simulink model "PAMtesting_draft1"  (R2023a)
settings: Solver=VariableStepAuto  StartTime=0.0  StopTime=inf  RelTol=1e-3
libraries: sldrtlib x4
settings Model: Creator=Siril TD  LastModifiedBy=Siril TD

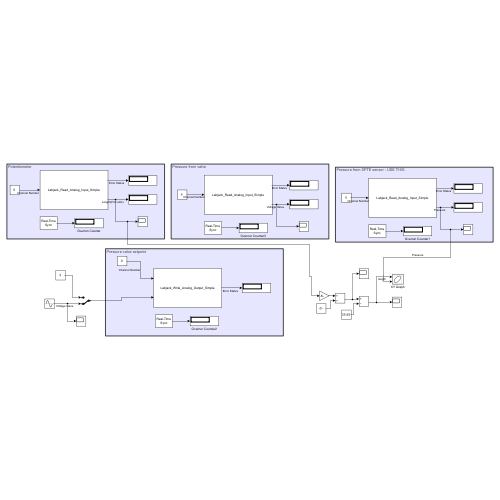
[thumbnail: Simulink's stored preview of the top-level diagram]
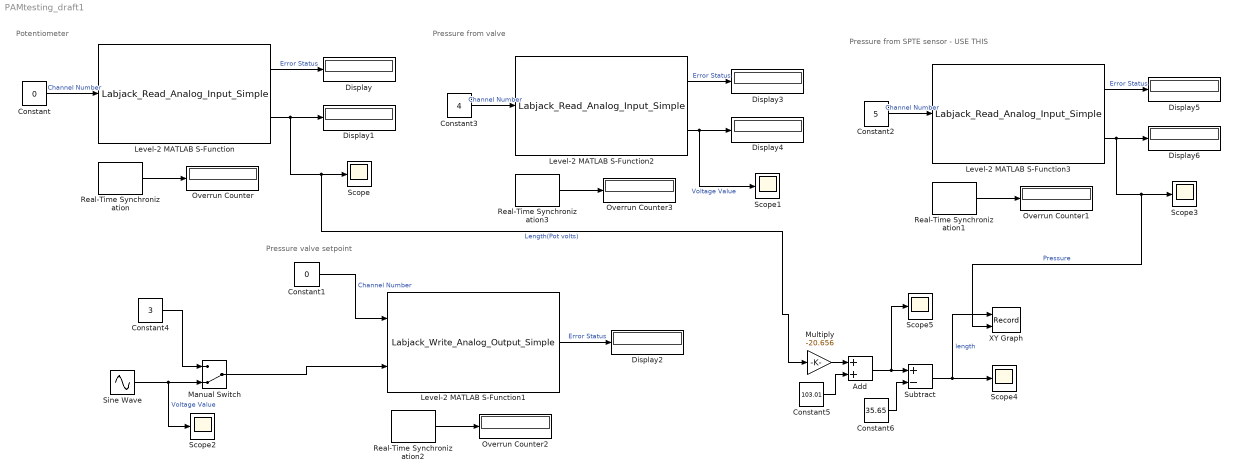
== system PAMtesting_draft1 ==
  note: Pressure valve setpoint
  note: Potentiometer
  note: Pressure from valve
  note: Pressure from SPTE sensor - USE THIS
  Add : Sum
  Constant : Constant  Value=0
  Constant1 : Constant  Value=0
  Constant2 : Constant  Value=5
  Constant3 : Constant  Value=4
  Constant4 : Constant  Value=3
  Constant5 : Constant  Value=103.01
  Constant6 : Constant  Value=35.65
  Display{,1..6} (7 alike) : Display
  Level-2 MATLAB S-Function : M-S-Function  FunctionName=Labjack_Read_Analog_Input_Simple
  Level-2 MATLAB S-Function1 : M-S-Function  FunctionName=Labjack_Write_Analog_Output_Simple
  Level-2 MATLAB S-Function2 : M-S-Function  FunctionName=Labjack_Read_Analog_Input_Simple
  Level-2 MATLAB S-Function3 : M-S-Function  FunctionName=Labjack_Read_Analog_Input_Simple
  Manual Switch : ManualSwitch  CurrentSetting=0
  Multiply : Gain  Gain=-20.656
  Overrun Counter{,1..3} (4 alike) : Display
  Real-Time Synchronization{,1..3} (4 alike) : sldrtlib/Real-Time Synchronization  SampleTime=0.1  MaxMissedTicks=100  ShowMissedTicks=on  YieldWhenWaiting=off
  Scope{,1..5} (6 alike) : Scope
  Sine Wave : Sin  Amplitude=2.5  Bias=2.5  Frequency=0.1  SampleTime=0
  Subtract : Sum  Inputs=+-
  XY Graph : Record  FileSettingsInternal="{\"entries\":[{\"content\":{\"excelSettings\":{\"content\":{},\"type\":\"Streamout.ExcelSettings\"}},\"type\":\"Streamout.FileSettingStorage\",\"uuid\":\"\"}],\"packageUris\":[\"http:\\/\\/schema.mathworks.com\\/mf0\\/streamout_blocks\\/R2020a\"],\"version\":\"1.0\"}"  Layout=[1 1]  SignalsInternal="{\"entries\":[{\"content\":{\"signals\":[{\"content\":{\"blockPath\":[],\"dimensions\":[1],\"domain\":\"\",\"lineColor\":\"#a2142f\",\"plots\":[1],\"port\":1,\"signalID\":17,\"signalName\":\"length\"},\"type\":\"RecordBlkView.Signal\",\"uuid\":\"\"},{\"content\":{\"blockPath\":[],\"dimensions\":[1],\"domain\":\"\",\"lineColor\":\"#139fff\",\"plots\":[1],\"port\":2,\"signalID\":20,\"signalName\":\"Pressure\"},\"type\":\"RecordBlkView.Signal\",\"uuid\":\"\"}]},\"type\":\"RecordBlkView.InputSignals\",\"uuid\":\"\"}],\"packageUris\":[\"http:\\/\\/schema.mathworks.com\\/mf0\\/streamout_blocks\\/R2020a\"],\"version\":\"1.0\"}"  VisualizationBindings="{\"xyplotplugin\":{\"info\":[{\"series\":[{\"bindingParametersList\":[{\"parameter\":\"X-Axis\",\"signalID\":17,\"signalName\":\"length\"},{\"parameter\":\"Y-Axis\",\"signalID\":20,\"signalName\":\"Pressure\"}],\"seriesID\":4338}],\"subplotID\":1}]}}"  CompatibilityTag=XY
  wires:
  Constant/1 -> Level-2 MATLAB S-Function/1  "Channel Number"
  Level-2 MATLAB S-Function/1 -> Display/1  "Error Status"
  Real-Time Synchronization/1 -> Overrun Counter/1
  Level-2 MATLAB S-Function/2 -> Multiply/1, Scope/1, Display1/1  "Length(Pot volts)"
  Sine Wave/1 -> Scope2/1, Manual Switch/2  "Voltage Value"
  Constant1/1 -> Level-2 MATLAB S-Function1/1  "Channel Number"
  Level-2 MATLAB S-Function1/1 -> Display2/1  "Error Status"
  Real-Time Synchronization2/1 -> Overrun Counter2/1
  Level-2 MATLAB S-Function2/1 -> Display3/1  "Error Status"
  Real-Time Synchronization3/1 -> Overrun Counter3/1
  Level-2 MATLAB S-Function2/2 -> Scope1/1, Display4/1  "Voltage Value"
  Constant3/1 -> Level-2 MATLAB S-Function2/1  "Channel Number"
  Real-Time Synchronization1/1 -> Overrun Counter1/1
  Constant2/1 -> Level-2 MATLAB S-Function3/1  "Channel Number"
  Level-2 MATLAB S-Function3/1 -> Display5/1  "Error Status"
  Level-2 MATLAB S-Function3/2 -> XY Graph/2, Scope3/1, Display6/1  "Pressure"
  Manual Switch/1 -> Level-2 MATLAB S-Function1/2
  Constant4/1 -> Manual Switch/1
  Multiply/1 -> Add/1
  Constant5/1 -> Add/2
  Add/1 -> Scope5/1, Subtract/1
  Subtract/1 -> XY Graph/1, Scope4/1  "length"
  Constant6/1 -> Subtract/2
